simulink model "dog_x_bit_true_2023a1"  (R2023b)
settings: Solver=ode45  StartTime=0.0  StopTime=1.5*lsim*Ts  MaxStep=1/f0/2  RelTol=1e-6
values from neighbouring files (symbols this model uses):
  ft = (bint-1)*fbin    [exe_DOG_X_bit_true_2023a.m]    (also in exe_DOG_X_integer_true_two_paths_5b.m)
  g1 = g1_ideal*1    (= 4)    [exe_DOG_X_bit_true_2023a.m]    (also in exe_DOG_X_integer_true_two_paths_5b.m)
  Kvco = f0    (= 99840000)    [exe_DOG_X_bit_true_2023a.m]    (also in exe_DOG_X_integer_true_two_paths_5b.m)
  lvl = Vfs*10^(Input_signal_dB/20)    (= 0.242661009508)    [exe_DOG_X_bit_true_2023a.m]    (also in exe_DOG_X_integer_true_two_paths_5b.m = 0.125892541179)
  Nbsv1 = Nbvco+4    (= 9)    [exe_DOG_X_bit_true_2023a.m]    (also in exe_DOG_X_integer_true_two_paths_5b.m)
  Nbsv2 = Nbsv1+Nbext    [exe_DOG_X_bit_true_2023a.m]    (also in exe_DOG_X_integer_true_two_paths_5b.m)
  pnoi = 10^(-(60)/10)*(Vfs^2/2)    (= 5e-07)    [exe_DOG_X_bit_true_2023a.m]    (also in exe_DOG_X_integer_true_two_paths_5b.m)
  T2 = 1/f2    (= 4.06901041667e-08)    [exe_DOG_X_bit_true_2023a.m]    (also in exe_DOG_X_integer_true_two_paths_5b.m)
  Ts = 1/fs    (= 3.25520833333e-07)    [exe_DOG_X_bit_true_2023a.m]    (also in exe_DOG_X_integer_true_two_paths_5b.m)
  Vfs = 1    [exe_DOG_X_bit_true_2023a.m]    (also in exe_DOG_X_integer_true_two_paths_5b.m)
undefined symbols (not defined in the file or in its folder): fa, fb
libraries: simulink_extras x86, simulink x8
(part 1 of 4)
settings Model: SimulationMode=accelerator  Creator=lhernandez  LastModifiedBy=Richi
settings DataIOCC: SaveOutput=off  SignalLogging=off  DSMLogging=off  SaveTime=off  ReturnWorkspaceOutputs=off

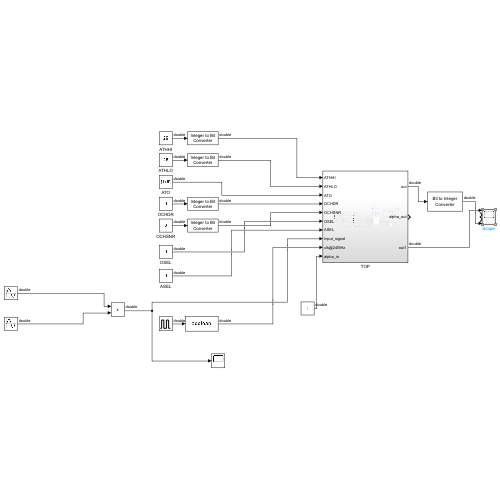
[thumbnail: Simulink's stored preview of the top-level diagram]
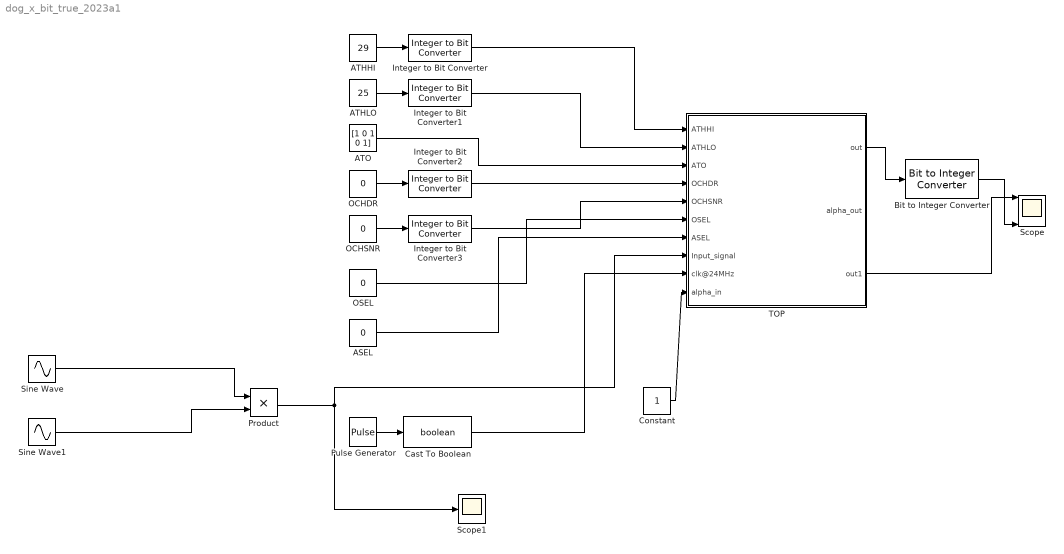
== system dog_x_bit_true_2023a1 ==
  ASEL : Constant  Value=0  OutDataTypeStr=boolean
  ATHHI : Constant  Value=29  OutDataTypeStr=fixdt(0,9,0)
  ATHLO : Constant  Value=25  OutDataTypeStr=fixdt(0,9,0)
  ATO : Constant  Value=[1 0 1 0 1]  OutDataTypeStr=boolean
  Bit to Integer Converter : simulink/Logic and Bit Operations/Bit to Integer Converter  nbits=11  bitOrder=MSB first  signedOutputValues=Signed  outDtype=Inherit via internal rule  outDtypeSigned=double
  Cast To Boolean : DataTypeConversion  OutDataTypeStr=boolean  SaturateOnIntegerOverflow=off  RndMeth=Floor
  Constant : Constant  OutDataTypeStr=boolean
  Integer to Bit Converter : simulink/Logic and Bit Operations/Integer to Bit Converter  nbits=9  signedInputValues=Unsigned  bitOrder=MSB first  outDtype=boolean
  Integer to Bit Converter1 : simulink/Logic and Bit Operations/Integer to Bit Converter  nbits=9  signedInputValues=Unsigned  bitOrder=MSB first  outDtype=boolean
  Integer to Bit Converter2 : simulink/Logic and Bit Operations/Integer to Bit Converter  nbits=4  signedInputValues=Signed  bitOrder=MSB first  outDtype=boolean
  Integer to Bit Converter3 : simulink/Logic and Bit Operations/Integer to Bit Converter  nbits=4  signedInputValues=Signed  bitOrder=MSB first  outDtype=boolean
  OCHDR : Constant  Value=0  OutDataTypeStr=fixdt(1,9,0)
  OCHSNR : Constant  Value=0  OutDataTypeStr=fixdt(1,9,0)
  OSEL : Constant  Value=0  OutDataTypeStr=boolean
  Product : Product
  Pulse Generator : DiscretePulseGenerator  PulseType=Time based  Period=T2  PulseWidth=50
  Scope : Scope  NumInputPorts=4
  Scope1 : Scope
  Sine Wave : Sin  Amplitude=lvl/Vfs  Frequency=2*pi*ft  SampleTime=0
  Sine Wave1 : Sin  Frequency=2*pi*250  SampleTime=0
  TOP : Subsystem
  wires:
  ATHHI/1 -> Integer to Bit Converter/1
  Integer to Bit Converter/1 -> TOP/1(ATHHI)
  ATHLO/1 -> Integer to Bit Converter1/1
  Integer to Bit Converter1/1 -> TOP/2(ATHLO)
  ATO/1 -> TOP/3(ATO)
  OCHDR/1 -> Integer to Bit Converter2/1
  Integer to Bit Converter2/1 -> TOP/4(OCHDR)
  OCHSNR/1 -> Integer to Bit Converter3/1
  Integer to Bit Converter3/1 -> TOP/5(OCHSNR)
  OSEL/1 -> TOP/6(OSEL)
  TOP/1(out) -> Bit to Integer Converter/1
  Pulse Generator/1 -> Cast To Boolean/1
  Cast To Boolean/1 -> TOP/9(clk@24MHz)
  ASEL/1 -> TOP/7(ASEL)
  Sine Wave1/1 -> Product/2
  Sine Wave/1 -> Product/1
  Product/1 -> TOP/8(Input_signal), Scope1/1
  Bit to Integer Converter/1 -> Scope/4
  Constant/1 -> TOP/10(alpha_in)
  TOP/3(out1) -> Scope/1

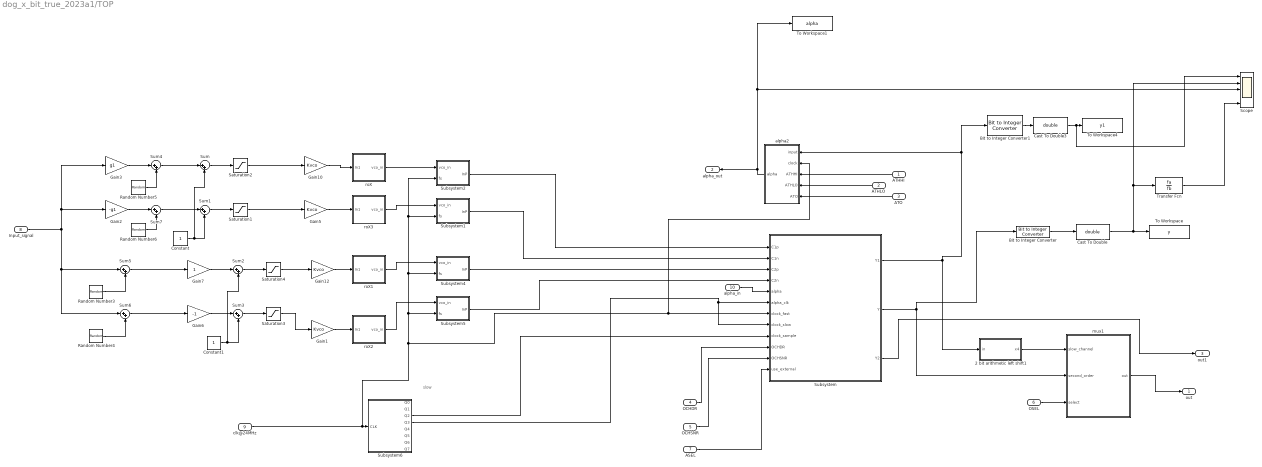
== system dog_x_bit_true_2023a1/TOP ==
  note: slow
  ATHHI : Inport
  ATHLO : Inport  Port=2
  ATO : Inport  Port=3
  OCHDR : Inport  Port=4
  OCHSNR : Inport  Port=5
  OSEL : Inport  Port=6
  ASEL : Inport  Port=7
  Input_signal : Inport  Port=8
  clk@24MHz : Inport  Port=9
  alpha_in : Inport  Port=10
  " 2 bit arithmetic left shift1" : Subsystem
  Bit to Integer Converter : simulink/Logic and Bit Operations/Bit to Integer Converter  nbits=11  bitOrder=MSB first  signedOutputValues=Signed  outDtype=Inherit via internal rule  outDtypeSigned=Inherit via internal rule
  Bit to Integer Converter1 : simulink/Logic and Bit Operations/Bit to Integer Converter  nbits=9  bitOrder=MSB first  signedOutputValues=Signed  outDtype=Inherit via internal rule  outDtypeSigned=Inherit via internal rule
  Cast To Double : DataTypeConversion  OutDataTypeStr=double  SaturateOnIntegerOverflow=off  RndMeth=Floor
  Cast To Double3 : DataTypeConversion  OutDataTypeStr=double  SaturateOnIntegerOverflow=off  RndMeth=Floor
  Constant : Constant
  Constant1 : Constant
  Gain{1,5,10,12} (4 alike) : Gain  Gain=Kvco
  Gain2 : Gain  Gain=-g1
  Gain3 : Gain  Gain=g1
  Gain6 : Gain  Gain=-1
  Gain7 : Gain
  Random Number3 : RandomNumber  Variance=pnoi  Seed=35645  SampleTime=0
  Random Number4 : RandomNumber  Variance=pnoi  Seed=6854  SampleTime=0
  Random Number5 : RandomNumber  Variance=pnoi  Seed=5747  SampleTime=0
  Random Number6 : RandomNumber  Variance=pnoi  Seed=254745  SampleTime=0
  Saturation{1..4} (4 alike) : Saturate  UpperLimit=2  LowerLimit=0
  Scope : Scope  NumInputPorts=5
  Subsystem : Subsystem
  Subsystem1 : Subsystem
  Subsystem2 : Subsystem
  Subsystem4 : Subsystem
  Subsystem5 : Subsystem
  Subsystem6 : Subsystem
  Sum{,1..7} (8 alike) : Sum  Inputs=|++
  To Workspace : ToWorkspace  VariableName=y  SampleTime=Ts
  To Workspace1 : ToWorkspace  VariableName=alpha  SampleTime=Ts
  To Workspace4 : ToWorkspace  VariableName=y1  SampleTime=Ts
  Transfer Fcn : TransferFcn  Numerator=fa  Denominator=fb
  alpha2 : Subsystem
  mux1 : Subsystem
  roX : Subsystem
  roX1 : Subsystem
  roX2 : Subsystem
  roX3 : Subsystem
  out : Outport
  alpha_out : Outport  Port=2
  out1 : Outport  Port=3
  wires:
  roX3/1(vco_in) -> Subsystem1/1(vco_in)
  ? -> Scope/4
  roX/1(vco_in) -> Subsystem2/1(vco_in)
  OSEL/1 -> mux1/3(select)
  ATHLO/1 -> alpha2/4(ATHLO)
  Random Number4/1 -> Sum6/2
  Gain7/1 -> Sum2/1
  Random Number6/1 -> Sum7/2
  Bit to Integer Converter1/1 -> Cast To Double3/1
  Random Number3/1 -> Sum5/2
  Cast To Double/1 -> Transfer Fcn/1, Scope/2, To Workspace/1
  Random Number5/1 -> Sum4/2
  Sum4/1 -> Sum/1
  Saturation4/1 -> Gain12/1
  Gain2/1 -> Sum7/1
  clk@24MHz/1 -> alpha2/2(clock), Subsystem/7(clock_fast), Subsystem5/2(fs), Subsystem4/2(fs), Subsystem2/2(fs), Subsystem1/2(fs), Subsystem6/1(CLK)
  Gain10/1 -> roX/1(In1)
  roX1/1(vco_in) -> Subsystem4/1(vco_in)
  Constant/1 -> Sum/2, Sum1/2
  Bit to Integer Converter/1 -> Cast To Double/1
  Gain3/1 -> Sum4/1
  Sum6/1 -> Gain6/1
  Transfer Fcn/1 -> Scope/5
  Gain5/1 -> roX3/1(In1)
  Sum7/1 -> Sum1/1
  roX2/1(vco_in) -> Subsystem5/1(vco_in)
  Sum/1 -> Saturation2/1
  Gain1/1 -> roX2/1(In1)
  Sum2/1 -> Saturation4/1
  mux1/1(out) -> out/1
  Constant1/1 -> Sum2/2, Sum3/2
  Saturation1/1 -> Gain5/1
  Subsystem/2(Y) -> mux1/2(second_order), Bit to Integer Converter/1
  Saturation3/1 -> Gain1/1
  Saturation2/1 -> Gain10/1
  Gain12/1 -> roX1/1(In1)
  alpha2/1(alpha) -> alpha_out/1, To Workspace1/1, Scope/3
  Cast To Double3/1 -> Scope/1, To Workspace4/1
  Gain6/1 -> Sum3/1
  Sum5/1 -> Gain7/1
  Subsystem/1(Y1) -> " 2 bit arithmetic left shift1"/1(in), Bit to Integer Converter1/1, alpha2/1(input)
  ATHHI/1 -> alpha2/3(ATHHI)
  Input_signal/1 -> Sum6/1, Sum5/1, Gain3/1, Gain2/1
  OCHSNR/1 -> Subsystem/11(OCHSNR)
  Sum3/1 -> Saturation3/1
  Sum1/1 -> Saturation1/1
  ATO/1 -> alpha2/5(ATO)
  OCHDR/1 -> Subsystem/10(OCHDR)
  " 2 bit arithmetic left shift1"/1(x4) -> mux1/1(slow_channel)
  Subsystem2/1(InP) -> Subsystem/1(C1p)
  Subsystem1/1(InP) -> Subsystem/2(C1n)
  Subsystem4/1(InP) -> Subsystem/3(C2p)
  Subsystem5/1(InP) -> Subsystem/4(C2n)
  Subsystem6/4(Q3) -> Subsystem/8(clock_slow), Subsystem/6(alpha_clk)
  Subsystem6/3(Q2) -> Subsystem/9(clock_sample)
  alpha_in/1 -> Subsystem/5(alpha)
  ASEL/1 -> Subsystem/12(use_external)
  Subsystem/3(Y2) -> out1/1

== system dog_x_bit_true_2023a1/TOP/ 2 bit arithmetic left shift1 ==
  in : Inport
  Constant : Constant  Value=0  OutDataTypeStr=boolean
  Demux1 : Demux  Outputs=9
  Mux : Mux  Inputs=11
  x4 : Outport
  wires:
  Mux/1 -> x4/1
  in/1 -> Demux1/1
  Demux1/1 -> Mux/1
  Demux1/2 -> Mux/2
  Demux1/3 -> Mux/3
  Demux1/4 -> Mux/4
  Demux1/5 -> Mux/5
  Demux1/6 -> Mux/6
  Demux1/7 -> Mux/7
  Demux1/8 -> Mux/8
  Demux1/9 -> Mux/9
  Constant/1 -> Mux/11, Mux/10

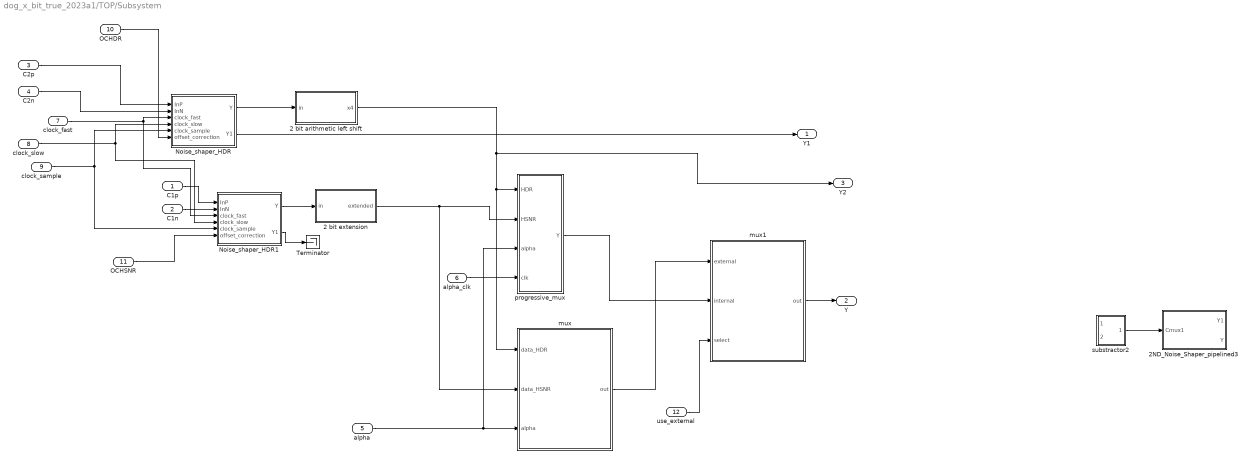
== system dog_x_bit_true_2023a1/TOP/Subsystem ==
  C1p : Inport
  C1n : Inport  Port=2
  C2p : Inport  Port=3
  C2n : Inport  Port=4
  alpha : Inport  Port=5
  alpha_clk : Inport  Port=6
  clock_fast : Inport  Port=7
  clock_slow : Inport  Port=8
  clock_sample : Inport  Port=9
  OCHDR : Inport  Port=10
  OCHSNR : Inport  Port=11
  use_external : Inport  Port=12
  " 2 bit arithmetic left shift" : Subsystem
  " 2 bit extension" : Subsystem
  2ND_Noise_Shaper_pipelined3 : Subsystem
  Noise_shaper_HDR : Subsystem
  Noise_shaper_HDR1 : Subsystem
  Terminator : Terminator
  mux : Subsystem
  mux1 : Subsystem
  progressive_mux : Subsystem
  substractor2 : Subsystem
  Y1 : Outport
  Y : Outport  Port=2
  Y2 : Outport  Port=3
  wires:
  substractor2/1(Cmux1) -> 2ND_Noise_Shaper_pipelined3/1(Cmux1)
  C2p/1 -> Noise_shaper_HDR/1(InP)
  C2n/1 -> Noise_shaper_HDR/2(InN)
  alpha_clk/1 -> progressive_mux/4(clk)
  clock_fast/1 -> Noise_shaper_HDR1/3(clock_fast), Noise_shaper_HDR/3(clock_fast)
  clock_slow/1 -> Noise_shaper_HDR1/4(clock_slow), Noise_shaper_HDR/4(clock_slow)
  Noise_shaper_HDR/1(Y) -> " 2 bit arithmetic left shift"/1(in)
  " 2 bit arithmetic left shift"/1(x4) -> Y2/1, progressive_mux/1(HDR), mux/1(data_HDR)
  clock_sample/1 -> Noise_shaper_HDR1/5(clock_sample), Noise_shaper_HDR/5(clock_sample)
  " 2 bit extension"/1(extended) -> progressive_mux/2(HSNR), mux/2(data_HSNR)
  C1n/1 -> Noise_shaper_HDR1/2(InN)
  C1p/1 -> Noise_shaper_HDR1/1(InP)
  Noise_shaper_HDR1/1(Y) -> " 2 bit extension"/1(in)
  Noise_shaper_HDR1/2(Y1) -> Terminator/1
  mux1/1(out) -> Y/1
  Noise_shaper_HDR/2(Y1) -> Y1/1
  use_external/1 -> mux1/3(select)
  mux/1(out) -> mux1/1(external)
  progressive_mux/1(Y) -> mux1/2(internal)
  alpha/1 -> progressive_mux/3(alpha), mux/3(alpha)
  OCHSNR/1 -> Noise_shaper_HDR1/6(offset_correction)
  OCHDR/1 -> Noise_shaper_HDR/6(offset_correction)

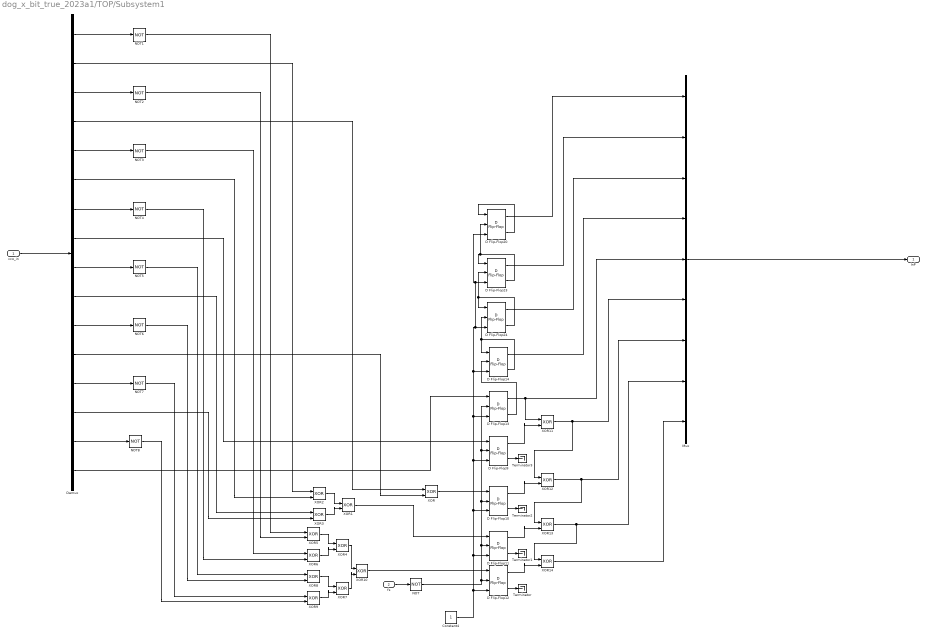
== system dog_x_bit_true_2023a1/TOP/Subsystem1 ==
  vco_in : Inport
  fs : Inport  Port=2
  Constant4 : Constant
  D Flip-Flop{9..14,20,23..24} (9 alike) : simulink_extras/Flip Flops/D Flip-Flop
  Demux : Demux  Outputs=16
  Mux : Mux  Inputs=9
  NOT{,1..8} (9 alike) : Logic  Operator=NOT  IconShape=distinctive  AllPortsSameDT=off  OutDataTypeStr=boolean
  Terminator{,1..3} (4 alike) : Terminator
  XOR{,1..14} (15 alike) : Logic  Operator=XOR  IconShape=distinctive  AllPortsSameDT=off  OutDataTypeStr=boolean
  InP : Outport
  wires:
  D Flip-Flop12/2 -> Terminator/1
  D Flip-Flop10/2 -> Terminator2/1
  D Flip-Flop11/2 -> Terminator1/1
  D Flip-Flop23/2 -> D Flip-Flop20/2, D Flip-Flop23/1
  D Flip-Flop24/2 -> D Flip-Flop24/1, D Flip-Flop23/2
  D Flip-Flop20/2 -> D Flip-Flop20/1
  fs/1 -> NOT/1
  D Flip-Flop14/2 -> D Flip-Flop14/1, D Flip-Flop24/2
  Mux/1 -> InP/1
  Constant4/1 -> D Flip-Flop12/3, D Flip-Flop11/3, D Flip-Flop10/3, D Flip-Flop20/3, D Flip-Flop23/3, D Flip-Flop24/3, D Flip-Flop14/3, D Flip-Flop13/3, D Flip-Flop9/3
  D Flip-Flop13/2 -> D Flip-Flop14/2
  NOT/1 -> D Flip-Flop12/2, D Flip-Flop13/2, D Flip-Flop9/2, D Flip-Flop10/2, D Flip-Flop11/2
  D Flip-Flop9/2 -> Terminator3/1
  vco_in/1 -> Demux/1
  Demux/1 -> NOT1/1
  Demux/5 -> NOT3/1
  Demux/7 -> NOT4/1
  Demux/9 -> NOT5/1
  Demux/13 -> NOT7/1
  Demux/15 -> NOT8/1
  Demux/11 -> NOT6/1
  Demux/4 -> XOR/1
  Demux/12 -> XOR/2
  XOR2/1 -> XOR1/1
  XOR3/1 -> XOR1/2
  Demux/2 -> XOR2/1
  Demux/6 -> XOR2/2
  Demux/10 -> XOR3/1
  Demux/14 -> XOR3/2
  XOR5/1 -> XOR4/1
  XOR6/1 -> XOR4/2
  XOR8/1 -> XOR7/1
  XOR9/1 -> XOR7/2
  XOR4/1 -> XOR10/1
  XOR7/1 -> XOR10/2
  Demux/3 -> NOT2/1
  D Flip-Flop13/1 -> Mux/5, XOR11/1
  D Flip-Flop9/1 -> XOR11/2
  XOR11/1 -> Mux/6, XOR12/1
  D Flip-Flop10/1 -> XOR12/2
  XOR12/1 -> Mux/7, XOR13/1
  D Flip-Flop11/1 -> XOR13/2
  XOR13/1 -> Mux/8, XOR14/1
  D Flip-Flop12/1 -> XOR14/2
  NOT1/1 -> XOR5/1
  NOT2/1 -> XOR5/2
  NOT3/1 -> XOR6/1
  NOT4/1 -> XOR6/2
  NOT5/1 -> XOR8/1
  NOT6/1 -> XOR8/2
  NOT7/1 -> XOR9/1
  NOT8/1 -> XOR9/2
  Demux/16 -> D Flip-Flop13/1
  Demux/8 -> D Flip-Flop9/1
  XOR/1 -> D Flip-Flop10/1
  XOR1/1 -> D Flip-Flop11/1
  XOR10/1 -> D Flip-Flop12/1
  XOR14/1 -> Mux/9
  D Flip-Flop14/1 -> Mux/4
  D Flip-Flop24/1 -> Mux/3
  D Flip-Flop23/1 -> Mux/2
  D Flip-Flop20/1 -> Mux/1

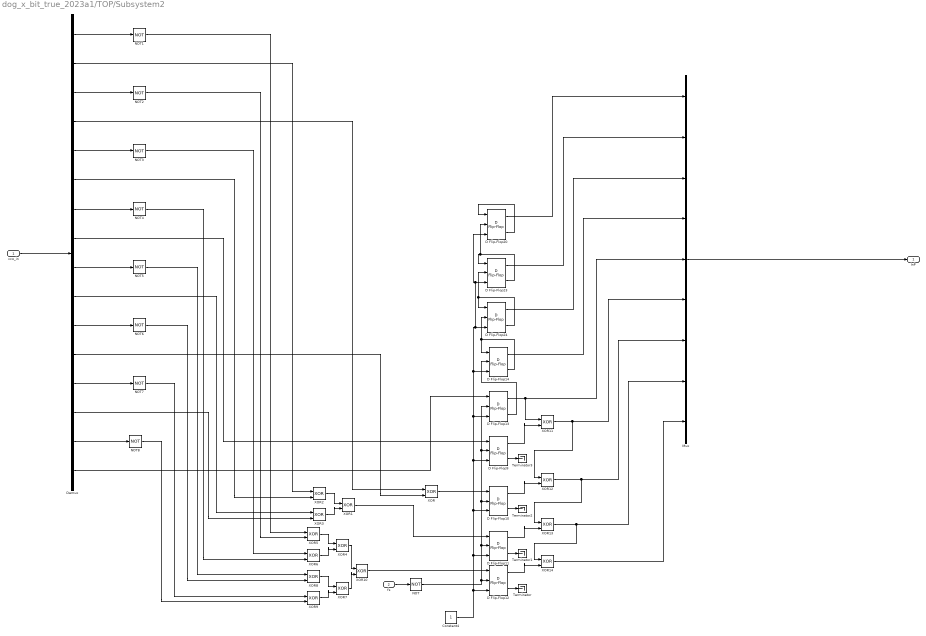
== system dog_x_bit_true_2023a1/TOP/Subsystem2 ==
  vco_in : Inport
  fs : Inport  Port=2
  Constant4 : Constant
  D Flip-Flop{9..14,20,23..24} (9 alike) : simulink_extras/Flip Flops/D Flip-Flop
  Demux : Demux  Outputs=16
  Mux : Mux  Inputs=9
  NOT{,1..8} (9 alike) : Logic  Operator=NOT  IconShape=distinctive  AllPortsSameDT=off  OutDataTypeStr=boolean
  Terminator{,1..3} (4 alike) : Terminator
  XOR{,1..14} (15 alike) : Logic  Operator=XOR  IconShape=distinctive  AllPortsSameDT=off  OutDataTypeStr=boolean
  InP : Outport
  wires:
  D Flip-Flop12/2 -> Terminator/1
  D Flip-Flop10/2 -> Terminator2/1
  D Flip-Flop11/2 -> Terminator1/1
  D Flip-Flop23/2 -> D Flip-Flop20/2, D Flip-Flop23/1
  D Flip-Flop24/2 -> D Flip-Flop24/1, D Flip-Flop23/2
  D Flip-Flop20/2 -> D Flip-Flop20/1
  fs/1 -> NOT/1
  D Flip-Flop14/2 -> D Flip-Flop14/1, D Flip-Flop24/2
  Mux/1 -> InP/1
  Constant4/1 -> D Flip-Flop12/3, D Flip-Flop11/3, D Flip-Flop10/3, D Flip-Flop20/3, D Flip-Flop23/3, D Flip-Flop24/3, D Flip-Flop14/3, D Flip-Flop13/3, D Flip-Flop9/3
  D Flip-Flop13/2 -> D Flip-Flop14/2
  NOT/1 -> D Flip-Flop12/2, D Flip-Flop13/2, D Flip-Flop9/2, D Flip-Flop10/2, D Flip-Flop11/2
  D Flip-Flop9/2 -> Terminator3/1
  vco_in/1 -> Demux/1
  Demux/1 -> NOT1/1
  Demux/5 -> NOT3/1
  Demux/7 -> NOT4/1
  Demux/9 -> NOT5/1
  Demux/13 -> NOT7/1
  Demux/15 -> NOT8/1
  Demux/11 -> NOT6/1
  Demux/4 -> XOR/1
  Demux/12 -> XOR/2
  XOR2/1 -> XOR1/1
  XOR3/1 -> XOR1/2
  Demux/2 -> XOR2/1
  Demux/6 -> XOR2/2
  Demux/10 -> XOR3/1
  Demux/14 -> XOR3/2
  XOR5/1 -> XOR4/1
  XOR6/1 -> XOR4/2
  XOR8/1 -> XOR7/1
  XOR9/1 -> XOR7/2
  XOR4/1 -> XOR10/1
  XOR7/1 -> XOR10/2
  Demux/3 -> NOT2/1
  D Flip-Flop13/1 -> Mux/5, XOR11/1
  D Flip-Flop9/1 -> XOR11/2
  XOR11/1 -> Mux/6, XOR12/1
  D Flip-Flop10/1 -> XOR12/2
  XOR12/1 -> Mux/7, XOR13/1
  D Flip-Flop11/1 -> XOR13/2
  XOR13/1 -> Mux/8, XOR14/1
  D Flip-Flop12/1 -> XOR14/2
  NOT1/1 -> XOR5/1
  NOT2/1 -> XOR5/2
  NOT3/1 -> XOR6/1
  NOT4/1 -> XOR6/2
  NOT5/1 -> XOR8/1
  NOT6/1 -> XOR8/2
  NOT7/1 -> XOR9/1
  NOT8/1 -> XOR9/2
  Demux/16 -> D Flip-Flop13/1
  Demux/8 -> D Flip-Flop9/1
  XOR/1 -> D Flip-Flop10/1
  XOR1/1 -> D Flip-Flop11/1
  XOR10/1 -> D Flip-Flop12/1
  XOR14/1 -> Mux/9
  D Flip-Flop14/1 -> Mux/4
  D Flip-Flop24/1 -> Mux/3
  D Flip-Flop23/1 -> Mux/2
  D Flip-Flop20/1 -> Mux/1

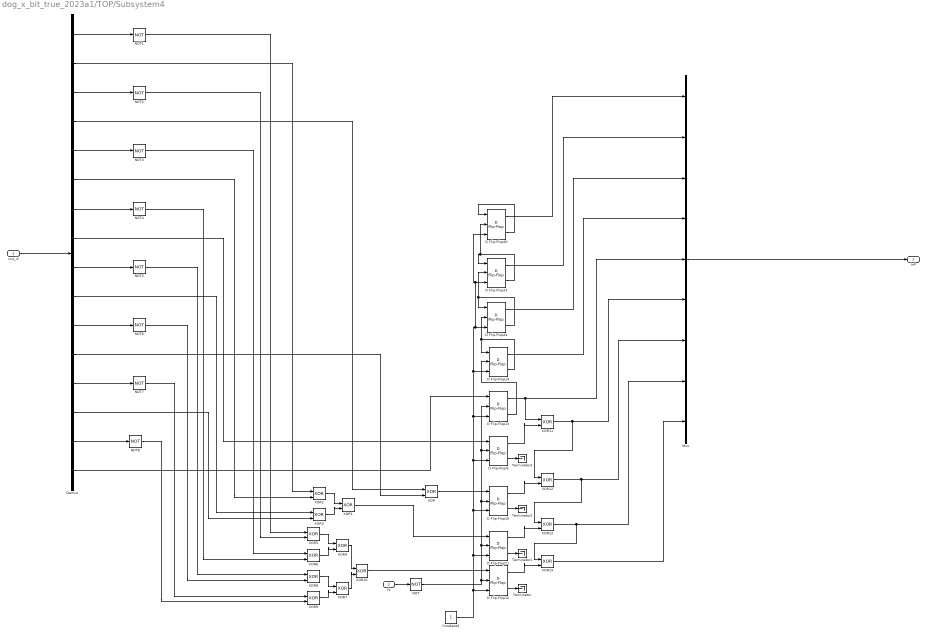
== system dog_x_bit_true_2023a1/TOP/Subsystem4 ==
  vco_in : Inport
  fs : Inport  Port=2
  Constant4 : Constant
  D Flip-Flop{9..14,20,23..24} (9 alike) : simulink_extras/Flip Flops/D Flip-Flop
  Demux : Demux  Outputs=16
  Mux : Mux  Inputs=9
  NOT{,1..8} (9 alike) : Logic  Operator=NOT  IconShape=distinctive  AllPortsSameDT=off  OutDataTypeStr=boolean
  Terminator{,1..3} (4 alike) : Terminator
  XOR{,1..14} (15 alike) : Logic  Operator=XOR  IconShape=distinctive  AllPortsSameDT=off  OutDataTypeStr=boolean
  InP : Outport
  wires:
  D Flip-Flop12/2 -> Terminator/1
  D Flip-Flop10/2 -> Terminator2/1
  D Flip-Flop11/2 -> Terminator1/1
  D Flip-Flop23/2 -> D Flip-Flop20/2, D Flip-Flop23/1
  D Flip-Flop24/2 -> D Flip-Flop24/1, D Flip-Flop23/2
  D Flip-Flop20/2 -> D Flip-Flop20/1
  fs/1 -> NOT/1
  D Flip-Flop14/2 -> D Flip-Flop14/1, D Flip-Flop24/2
  Mux/1 -> InP/1
  Constant4/1 -> D Flip-Flop12/3, D Flip-Flop11/3, D Flip-Flop10/3, D Flip-Flop20/3, D Flip-Flop23/3, D Flip-Flop24/3, D Flip-Flop14/3, D Flip-Flop13/3, D Flip-Flop9/3
  D Flip-Flop13/2 -> D Flip-Flop14/2
  NOT/1 -> D Flip-Flop12/2, D Flip-Flop13/2, D Flip-Flop9/2, D Flip-Flop10/2, D Flip-Flop11/2
  D Flip-Flop9/2 -> Terminator3/1
  vco_in/1 -> Demux/1
  Demux/1 -> NOT1/1
  Demux/5 -> NOT3/1
  Demux/7 -> NOT4/1
  Demux/9 -> NOT5/1
  Demux/13 -> NOT7/1
  Demux/15 -> NOT8/1
  Demux/11 -> NOT6/1
  Demux/4 -> XOR/1
  Demux/12 -> XOR/2
  XOR2/1 -> XOR1/1
  XOR3/1 -> XOR1/2
  Demux/2 -> XOR2/1
  Demux/6 -> XOR2/2
  Demux/10 -> XOR3/1
  Demux/14 -> XOR3/2
  XOR5/1 -> XOR4/1
  XOR6/1 -> XOR4/2
  XOR8/1 -> XOR7/1
  XOR9/1 -> XOR7/2
  XOR4/1 -> XOR10/1
  XOR7/1 -> XOR10/2
  Demux/3 -> NOT2/1
  D Flip-Flop13/1 -> Mux/5, XOR11/1
  D Flip-Flop9/1 -> XOR11/2
  XOR11/1 -> Mux/6, XOR12/1
  D Flip-Flop10/1 -> XOR12/2
  XOR12/1 -> Mux/7, XOR13/1
  D Flip-Flop11/1 -> XOR13/2
  XOR13/1 -> Mux/8, XOR14/1
  D Flip-Flop12/1 -> XOR14/2
  NOT1/1 -> XOR5/1
  NOT2/1 -> XOR5/2
  NOT3/1 -> XOR6/1
  NOT4/1 -> XOR6/2
  NOT5/1 -> XOR8/1
  NOT6/1 -> XOR8/2
  NOT7/1 -> XOR9/1
  NOT8/1 -> XOR9/2
  Demux/16 -> D Flip-Flop13/1
  Demux/8 -> D Flip-Flop9/1
  XOR/1 -> D Flip-Flop10/1
  XOR1/1 -> D Flip-Flop11/1
  XOR10/1 -> D Flip-Flop12/1
  XOR14/1 -> Mux/9
  D Flip-Flop14/1 -> Mux/4
  D Flip-Flop24/1 -> Mux/3
  D Flip-Flop23/1 -> Mux/2
  D Flip-Flop20/1 -> Mux/1

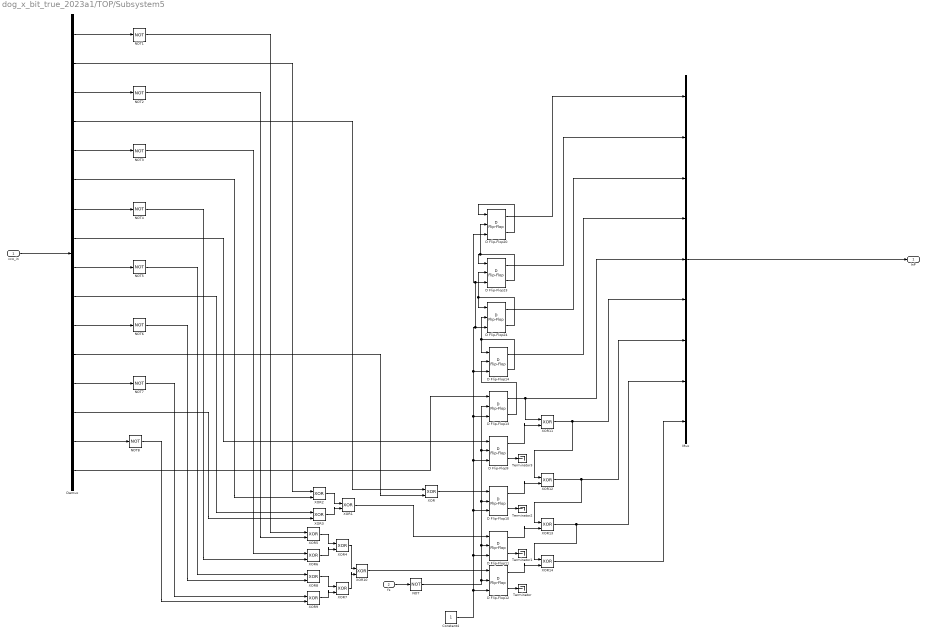
== system dog_x_bit_true_2023a1/TOP/Subsystem5 ==
  vco_in : Inport
  fs : Inport  Port=2
  Constant4 : Constant
  D Flip-Flop{9..14,20,23..24} (9 alike) : simulink_extras/Flip Flops/D Flip-Flop
  Demux : Demux  Outputs=16
  Mux : Mux  Inputs=9
  NOT{,1..8} (9 alike) : Logic  Operator=NOT  IconShape=distinctive  AllPortsSameDT=off  OutDataTypeStr=boolean
  Terminator{,1..3} (4 alike) : Terminator
  XOR{,1..14} (15 alike) : Logic  Operator=XOR  IconShape=distinctive  AllPortsSameDT=off  OutDataTypeStr=boolean
  InP : Outport
  wires:
  D Flip-Flop12/2 -> Terminator/1
  D Flip-Flop10/2 -> Terminator2/1
  D Flip-Flop11/2 -> Terminator1/1
  D Flip-Flop23/2 -> D Flip-Flop20/2, D Flip-Flop23/1
  D Flip-Flop24/2 -> D Flip-Flop24/1, D Flip-Flop23/2
  D Flip-Flop20/2 -> D Flip-Flop20/1
  fs/1 -> NOT/1
  D Flip-Flop14/2 -> D Flip-Flop14/1, D Flip-Flop24/2
  Mux/1 -> InP/1
  Constant4/1 -> D Flip-Flop12/3, D Flip-Flop11/3, D Flip-Flop10/3, D Flip-Flop20/3, D Flip-Flop23/3, D Flip-Flop24/3, D Flip-Flop14/3, D Flip-Flop13/3, D Flip-Flop9/3
  D Flip-Flop13/2 -> D Flip-Flop14/2
  NOT/1 -> D Flip-Flop12/2, D Flip-Flop13/2, D Flip-Flop9/2, D Flip-Flop10/2, D Flip-Flop11/2
  D Flip-Flop9/2 -> Terminator3/1
  vco_in/1 -> Demux/1
  Demux/1 -> NOT1/1
  Demux/5 -> NOT3/1
  Demux/7 -> NOT4/1
  Demux/9 -> NOT5/1
  Demux/13 -> NOT7/1
  Demux/15 -> NOT8/1
  Demux/11 -> NOT6/1
  Demux/4 -> XOR/1
  Demux/12 -> XOR/2
  XOR2/1 -> XOR1/1
  XOR3/1 -> XOR1/2
  Demux/2 -> XOR2/1
  Demux/6 -> XOR2/2
  Demux/10 -> XOR3/1
  Demux/14 -> XOR3/2
  XOR5/1 -> XOR4/1
  XOR6/1 -> XOR4/2
  XOR8/1 -> XOR7/1
  XOR9/1 -> XOR7/2
  XOR4/1 -> XOR10/1
  XOR7/1 -> XOR10/2
  Demux/3 -> NOT2/1
  D Flip-Flop13/1 -> Mux/5, XOR11/1
  D Flip-Flop9/1 -> XOR11/2
  XOR11/1 -> Mux/6, XOR12/1
  D Flip-Flop10/1 -> XOR12/2
  XOR12/1 -> Mux/7, XOR13/1
  D Flip-Flop11/1 -> XOR13/2
  XOR13/1 -> Mux/8, XOR14/1
  D Flip-Flop12/1 -> XOR14/2
  NOT1/1 -> XOR5/1
  NOT2/1 -> XOR5/2
  NOT3/1 -> XOR6/1
  NOT4/1 -> XOR6/2
  NOT5/1 -> XOR8/1
  NOT6/1 -> XOR8/2
  NOT7/1 -> XOR9/1
  NOT8/1 -> XOR9/2
  Demux/16 -> D Flip-Flop13/1
  Demux/8 -> D Flip-Flop9/1
  XOR/1 -> D Flip-Flop10/1
  XOR1/1 -> D Flip-Flop11/1
  XOR10/1 -> D Flip-Flop12/1
  XOR14/1 -> Mux/9
  D Flip-Flop14/1 -> Mux/4
  D Flip-Flop24/1 -> Mux/3
  D Flip-Flop23/1 -> Mux/2
  D Flip-Flop20/1 -> Mux/1

== system dog_x_bit_true_2023a1/TOP/Subsystem6 ==
  CLK : Inport
  Constant2 : Constant
  D Flip-Flop{,1..7} (8 alike) : simulink_extras/Flip Flops/D Flip-Flop
  Q0 : Outport
  Q1 : Outport  Port=2
  Q2 : Outport  Port=3
  Q3 : Outport  Port=4
  Q4 : Outport  Port=5
  Q5 : Outport  Port=6
  Q6 : Outport  Port=7
  Q7 : Outport  Port=8
  wires:
  D Flip-Flop2/2 -> D Flip-Flop3/2, D Flip-Flop2/1
  D Flip-Flop/2 -> D Flip-Flop1/2, D Flip-Flop/1
  D Flip-Flop2/1 -> Q2/1
  D Flip-Flop3/1 -> Q3/1
  D Flip-Flop/1 -> Q0/1
  D Flip-Flop1/1 -> Q1/1
  D Flip-Flop3/2 -> D Flip-Flop3/1, D Flip-Flop4/2
  D Flip-Flop1/2 -> D Flip-Flop2/2, D Flip-Flop1/1
  CLK/1 -> D Flip-Flop/2
  D Flip-Flop5/2 -> D Flip-Flop6/2, D Flip-Flop5/1
  D Flip-Flop4/1 -> Q4/1
  D Flip-Flop5/1 -> Q5/1
  Constant2/1 -> D Flip-Flop1/3, D Flip-Flop2/3, D Flip-Flop3/3, D Flip-Flop4/3, D Flip-Flop5/3, D Flip-Flop6/3, D Flip-Flop7/3, D Flip-Flop/3
  D Flip-Flop6/1 -> Q6/1
  D Flip-Flop7/2 -> D Flip-Flop7/1
  D Flip-Flop6/2 -> D Flip-Flop7/2, D Flip-Flop6/1
  D Flip-Flop7/1 -> Q7/1
  D Flip-Flop4/2 -> D Flip-Flop5/2, D Flip-Flop4/1

== system dog_x_bit_true_2023a1/TOP/alpha2 ==
  note: si a > b, reset
  note: si a > b, HDR
  input : Inport
  clock : Inport  Port=2
  ATHHI : Inport  Port=3
  ATHLO : Inport  Port=4
  ATO : Inport  Port=5
  10 bit  counter (pos) : Subsystem
  AND : Logic  IconShape=distinctive  AllPortsSameDT=off  OutDataTypeStr=boolean
  AND1 : Logic  IconShape=distinctive  AllPortsSameDT=off  OutDataTypeStr=boolean
  NOT : Logic  Operator=NOT  IconShape=distinctive  AllPortsSameDT=off  OutDataTypeStr=boolean
  NOT1 : Logic  Operator=NOT  IconShape=distinctive  AllPortsSameDT=off  OutDataTypeStr=boolean
  NOT2 : Logic  Operator=NOT  IconShape=distinctive  AllPortsSameDT=off  OutDataTypeStr=boolean
  S-R Flip-Flop : simulink_extras/Flip Flops/S-R Flip-Flop  initial_condition=0
  Terminator : Terminator
  abs : Subsystem
  comp_HI_Threshold : Subsystem
  comp_LOW_Threshold : Subsystem
  alpha : Outport
  wires:
  input/1 -> abs/1(input)
  S-R Flip-Flop/1 -> alpha/1
  clock/1 -> 10 bit  counter (pos)/2(clock)
  ATHLO/1 -> comp_LOW_Threshold/2(b)
  NOT1/1 -> 10 bit  counter (pos)/3(!reset)
  abs/1(abs(input)) -> comp_HI_Threshold/1(a), comp_LOW_Threshold/1(a)
  ATHHI/1 -> comp_HI_Threshold/2(b)
  S-R Flip-Flop/2 -> Terminator/1
  comp_LOW_Threshold/1(a < b) -> AND/2
  AND1/1 -> S-R Flip-Flop/2
  comp_HI_Threshold/1(a > b) -> NOT1/1, NOT2/1, S-R Flip-Flop/1
  NOT/1 -> AND/1
  NOT2/1 -> AND1/1
  10 bit  counter (pos)/1(count_selected_bit) -> AND1/2, NOT/1
  AND/1 -> 10 bit  counter (pos)/1(count_enable)
  ATO/1 -> 10 bit  counter (pos)/4(bit_select_mask)

== system dog_x_bit_true_2023a1/TOP/mux1 ==
  slow_channel : Inport
  second_order : Inport  Port=2
  select : Inport  Port=3
  Demux : Demux  Outputs=11
  Demux1 : Demux  Outputs=11
  Mux : Mux  Inputs=11
  Switch{,1..10} (11 alike) : Switch  Criteria=u2 > Threshold  SaturateOnIntegerOverflow=off  InputSameDT=off
  out : Outport
  wires:
  select/1 -> Switch1/2, Switch2/2, Switch3/2, Switch4/2, Switch6/2, Switch7/2, Switch8/2, Switch9/2, Switch10/2, Switch5/2, Switch/2
  slow_channel/1 -> Demux/1
  second_order/1 -> Demux1/1
  Demux/1 -> Switch/1
  Mux/1 -> out/1
  Demux/2 -> Switch1/1
  Demux/3 -> Switch2/1
  Demux/4 -> Switch3/1
  Demux/5 -> Switch4/1
  Demux/6 -> Switch5/1
  Demux/7 -> Switch6/1
  Demux/8 -> Switch7/1
  Demux/9 -> Switch8/1
  Demux/10 -> Switch9/1
  Demux/11 -> Switch10/1
  Demux1/1 -> Switch/3
  Demux1/2 -> Switch1/3
  Demux1/3 -> Switch2/3
  Demux1/4 -> Switch3/3
  Demux1/5 -> Switch4/3
  Demux1/6 -> Switch5/3
  Demux1/7 -> Switch6/3
  Demux1/8 -> Switch7/3
  Demux1/9 -> Switch8/3
  Demux1/10 -> Switch9/3
  Demux1/11 -> Switch10/3
  Switch/1 -> Mux/1
  Switch1/1 -> Mux/2
  Switch2/1 -> Mux/3
  Switch3/1 -> Mux/4
  Switch4/1 -> Mux/5
  Switch5/1 -> Mux/6
  Switch6/1 -> Mux/7
  Switch7/1 -> Mux/8
  Switch8/1 -> Mux/9
  Switch9/1 -> Mux/10
  Switch10/1 -> Mux/11

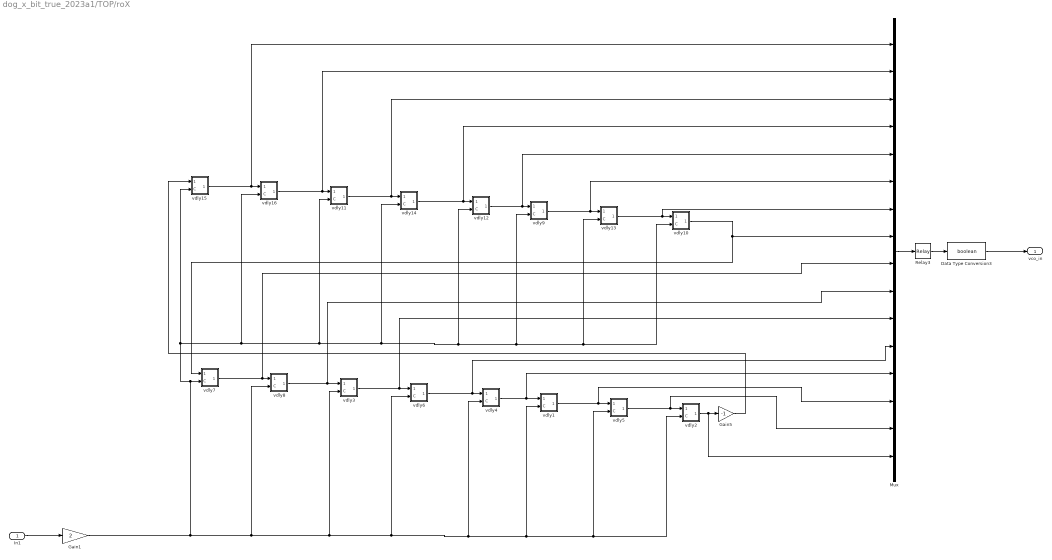
== system dog_x_bit_true_2023a1/TOP/roX ==
  In1 : Inport
  Data Type Conversion3 : DataTypeConversion  OutDataTypeStr=boolean  SaturateOnIntegerOverflow=off  RndMeth=Floor
  Gain1 : Gain  Gain=2
  Gain5 : Gain  Gain=-1
  Mux : Mux  Inputs=16
  Relay3 : Relay
  vdly1 : Subsystem
  vdly10 : Subsystem
  vdly11 : Subsystem
  vdly12 : Subsystem
  vdly13 : Subsystem
  vdly14 : Subsystem
  vdly15 : Subsystem
  vdly16 : Subsystem
  vdly2 : Subsystem
  vdly3 : Subsystem
  vdly4 : Subsystem
  vdly5 : Subsystem
  vdly6 : Subsystem
  vdly7 : Subsystem
  vdly8 : Subsystem
  vdly9 : Subsystem
  vco_in : Outport
  wires:
  vdly2/1(Out) -> Mux/16, Gain5/1
  In1/1 -> Gain1/1
  Gain1/1 -> vdly15/2(C), vdly16/2(C), vdly11/2(C), vdly14/2(C), vdly12/2(C), vdly9/2(C), vdly10/2(C), vdly13/2(C), vdly7/2(C), vdly8/2(C), vdly3/2(C), vdly6/2(C), vdly4/2(C), vdly1/2(C), vdly2/2(C), vdly5/2(C)
  Gain5/1 -> vdly15/1(In)
  Mux/1 -> Relay3/1
  Relay3/1 -> Data Type Conversion3/1
  Data Type Conversion3/1 -> vco_in/1
  vdly5/1(Out) -> Mux/15, vdly2/1(In)
  vdly1/1(Out) -> Mux/14, vdly5/1(In)
  vdly4/1(Out) -> Mux/13, vdly1/1(In)
  vdly6/1(Out) -> Mux/12, vdly4/1(In)
  vdly3/1(Out) -> Mux/11, vdly6/1(In)
  vdly8/1(Out) -> Mux/10, vdly3/1(In)
  vdly7/1(Out) -> vdly8/1(In), Mux/9
  vdly15/1(Out) -> Mux/1, vdly16/1(In)
  vdly16/1(Out) -> Mux/2, vdly11/1(In)
  vdly11/1(Out) -> Mux/3, vdly14/1(In)
  vdly14/1(Out) -> Mux/4, vdly12/1(In)
  vdly12/1(Out) -> Mux/5, vdly9/1(In)
  vdly9/1(Out) -> Mux/6, vdly13/1(In)
  vdly13/1(Out) -> Mux/7, vdly10/1(In)
  vdly10/1(Out) -> vdly7/1(In), Mux/8

== system dog_x_bit_true_2023a1/TOP/roX1 ==
  In1 : Inport
  Data Type Conversion3 : DataTypeConversion  OutDataTypeStr=boolean  SaturateOnIntegerOverflow=off  RndMeth=Floor
  Gain1 : Gain  Gain=2
  Gain5 : Gain  Gain=-1
  Mux : Mux  Inputs=16
  Relay3 : Relay
  vdly1 : Subsystem
  vdly10 : Subsystem
  vdly11 : Subsystem
  vdly12 : Subsystem
  vdly13 : Subsystem
  vdly14 : Subsystem
  vdly15 : Subsystem
  vdly16 : Subsystem
  vdly2 : Subsystem
  vdly3 : Subsystem
  vdly4 : Subsystem
  vdly5 : Subsystem
  vdly6 : Subsystem
  vdly7 : Subsystem
  vdly8 : Subsystem
  vdly9 : Subsystem
  vco_in : Outport
  wires:
  vdly2/1(Out) -> Mux/16, Gain5/1
  In1/1 -> Gain1/1
  Gain1/1 -> vdly15/2(C), vdly16/2(C), vdly11/2(C), vdly14/2(C), vdly12/2(C), vdly9/2(C), vdly10/2(C), vdly13/2(C), vdly7/2(C), vdly8/2(C), vdly3/2(C), vdly6/2(C), vdly4/2(C), vdly1/2(C), vdly2/2(C), vdly5/2(C)
  Gain5/1 -> vdly15/1(In)
  Mux/1 -> Relay3/1
  Relay3/1 -> Data Type Conversion3/1
  Data Type Conversion3/1 -> vco_in/1
  vdly5/1(Out) -> Mux/15, vdly2/1(In)
  vdly1/1(Out) -> Mux/14, vdly5/1(In)
  vdly4/1(Out) -> Mux/13, vdly1/1(In)
  vdly6/1(Out) -> Mux/12, vdly4/1(In)
  vdly3/1(Out) -> Mux/11, vdly6/1(In)
  vdly8/1(Out) -> Mux/10, vdly3/1(In)
  vdly7/1(Out) -> vdly8/1(In), Mux/9
  vdly15/1(Out) -> Mux/1, vdly16/1(In)
  vdly16/1(Out) -> Mux/2, vdly11/1(In)
  vdly11/1(Out) -> Mux/3, vdly14/1(In)
  vdly14/1(Out) -> Mux/4, vdly12/1(In)
  vdly12/1(Out) -> Mux/5, vdly9/1(In)
  vdly9/1(Out) -> Mux/6, vdly13/1(In)
  vdly13/1(Out) -> Mux/7, vdly10/1(In)
  vdly10/1(Out) -> vdly7/1(In), Mux/8

== system dog_x_bit_true_2023a1/TOP/roX2 ==
  In1 : Inport
  Data Type Conversion3 : DataTypeConversion  OutDataTypeStr=boolean  SaturateOnIntegerOverflow=off  RndMeth=Floor
  Gain1 : Gain  Gain=2
  Gain5 : Gain  Gain=-1
  Mux : Mux  Inputs=16
  Relay3 : Relay
  vdly1 : Subsystem
  vdly10 : Subsystem
  vdly11 : Subsystem
  vdly12 : Subsystem
  vdly13 : Subsystem
  vdly14 : Subsystem
  vdly15 : Subsystem
  vdly16 : Subsystem
  vdly2 : Subsystem
  vdly3 : Subsystem
  vdly4 : Subsystem
  vdly5 : Subsystem
  vdly6 : Subsystem
  vdly7 : Subsystem
  vdly8 : Subsystem
  vdly9 : Subsystem
  vco_in : Outport
  wires:
  vdly2/1(Out) -> Mux/16, Gain5/1
  In1/1 -> Gain1/1
  Gain1/1 -> vdly15/2(C), vdly16/2(C), vdly11/2(C), vdly14/2(C), vdly12/2(C), vdly9/2(C), vdly10/2(C), vdly13/2(C), vdly7/2(C), vdly8/2(C), vdly3/2(C), vdly6/2(C), vdly4/2(C), vdly1/2(C), vdly2/2(C), vdly5/2(C)
  Gain5/1 -> vdly15/1(In)
  Mux/1 -> Relay3/1
  Relay3/1 -> Data Type Conversion3/1
  Data Type Conversion3/1 -> vco_in/1
  vdly5/1(Out) -> Mux/15, vdly2/1(In)
  vdly1/1(Out) -> Mux/14, vdly5/1(In)
  vdly4/1(Out) -> Mux/13, vdly1/1(In)
  vdly6/1(Out) -> Mux/12, vdly4/1(In)
  vdly3/1(Out) -> Mux/11, vdly6/1(In)
  vdly8/1(Out) -> Mux/10, vdly3/1(In)
  vdly7/1(Out) -> vdly8/1(In), Mux/9
  vdly15/1(Out) -> Mux/1, vdly16/1(In)
  vdly16/1(Out) -> Mux/2, vdly11/1(In)
  vdly11/1(Out) -> Mux/3, vdly14/1(In)
  vdly14/1(Out) -> Mux/4, vdly12/1(In)
  vdly12/1(Out) -> Mux/5, vdly9/1(In)
  vdly9/1(Out) -> Mux/6, vdly13/1(In)
  vdly13/1(Out) -> Mux/7, vdly10/1(In)
  vdly10/1(Out) -> vdly7/1(In), Mux/8

== system dog_x_bit_true_2023a1/TOP/roX3 ==
  In1 : Inport
  Data Type Conversion3 : DataTypeConversion  OutDataTypeStr=boolean  SaturateOnIntegerOverflow=off  RndMeth=Floor
  Gain1 : Gain  Gain=2
  Gain5 : Gain  Gain=-1
  Mux : Mux  Inputs=16
  Relay3 : Relay
  vdly1 : Subsystem
  vdly10 : Subsystem
  vdly11 : Subsystem
  vdly12 : Subsystem
  vdly13 : Subsystem
  vdly14 : Subsystem
  vdly15 : Subsystem
  vdly16 : Subsystem
  vdly2 : Subsystem
  vdly3 : Subsystem
  vdly4 : Subsystem
  vdly5 : Subsystem
  vdly6 : Subsystem
  vdly7 : Subsystem
  vdly8 : Subsystem
  vdly9 : Subsystem
  vco_in : Outport
  wires:
  vdly2/1(Out) -> Mux/16, Gain5/1
  In1/1 -> Gain1/1
  Gain1/1 -> vdly15/2(C), vdly16/2(C), vdly11/2(C), vdly14/2(C), vdly12/2(C), vdly9/2(C), vdly10/2(C), vdly13/2(C), vdly7/2(C), vdly8/2(C), vdly3/2(C), vdly6/2(C), vdly4/2(C), vdly1/2(C), vdly2/2(C), vdly5/2(C)
  Gain5/1 -> vdly15/1(In)
  Mux/1 -> Relay3/1
  Relay3/1 -> Data Type Conversion3/1
  Data Type Conversion3/1 -> vco_in/1
  vdly5/1(Out) -> Mux/15, vdly2/1(In)
  vdly1/1(Out) -> Mux/14, vdly5/1(In)
  vdly4/1(Out) -> Mux/13, vdly1/1(In)
  vdly6/1(Out) -> Mux/12, vdly4/1(In)
  vdly3/1(Out) -> Mux/11, vdly6/1(In)
  vdly8/1(Out) -> Mux/10, vdly3/1(In)
  vdly7/1(Out) -> vdly8/1(In), Mux/9
  vdly15/1(Out) -> Mux/1, vdly16/1(In)
  vdly16/1(Out) -> Mux/2, vdly11/1(In)
  vdly11/1(Out) -> Mux/3, vdly14/1(In)
  vdly14/1(Out) -> Mux/4, vdly12/1(In)
  vdly12/1(Out) -> Mux/5, vdly9/1(In)
  vdly9/1(Out) -> Mux/6, vdly13/1(In)
  vdly13/1(Out) -> Mux/7, vdly10/1(In)
  vdly10/1(Out) -> vdly7/1(In), Mux/8

== system dog_x_bit_true_2023a1/TOP/Subsystem/ 2 bit arithmetic left shift ==
  in : Inport
  Constant : Constant  Value=0  OutDataTypeStr=boolean
  Demux1 : Demux  Outputs=9
  Mux : Mux  Inputs=11
  x4 : Outport
  wires:
  Mux/1 -> x4/1
  in/1 -> Demux1/1
  Demux1/1 -> Mux/1
  Demux1/2 -> Mux/2
  Demux1/3 -> Mux/3
  Demux1/4 -> Mux/4
  Demux1/5 -> Mux/5
  Demux1/6 -> Mux/6
  Demux1/7 -> Mux/7
  Demux1/8 -> Mux/8
  Demux1/9 -> Mux/9
  Constant/1 -> Mux/11, Mux/10

== system dog_x_bit_true_2023a1/TOP/Subsystem/ 2 bit extension ==
  in : Inport
  Demux1 : Demux  Outputs=9
  Mux : Mux  Inputs=11
  extended : Outport
  wires:
  Mux/1 -> extended/1
  in/1 -> Demux1/1
  Demux1/1 -> Mux/3, Mux/2, Mux/1
  Demux1/2 -> Mux/4
  Demux1/3 -> Mux/5
  Demux1/4 -> Mux/6
  Demux1/5 -> Mux/7
  Demux1/6 -> Mux/8
  Demux1/7 -> Mux/9
  Demux1/8 -> Mux/10
  Demux1/9 -> Mux/11

== system dog_x_bit_true_2023a1/TOP/Subsystem/2ND_Noise_Shaper_pipelined3 ==
  note: 1 / (2^n_shift)
  Cmux1 : Inport
  Data Type Conversion1 : DataTypeConversion  OutDataTypeStr=fixdt(1,Nbsv2,0)  SaturateOnIntegerOverflow=off  RndMeth=Floor
  Data Type Conversion2 : DataTypeConversion  OutDataTypeStr=fixdt(1,Nbsv2,0)  SaturateOnIntegerOverflow=off  RndMeth=Floor
  Delay4 : Delay  DelayLength=1  SampleTime=Ts
  Gain11 : Gain  Gain=1/2^(Nbsv2-Nbsv1)  OutDataTypeStr=fixdt(1,Nbsv1,0)
  M3 : Delay  DelayLength=1  SampleTime=T2
  M4 : Delay  DelayLength=1  SampleTime=T2
  M5 : ZeroOrderHold  SampleTime=Ts
  Sum20 : Sum  Inputs=|+-  OutDataTypeStr=fixdt(1,Nbsv1,0)
  Sum22 : Sum  Inputs=|+-  OutDataTypeStr=fixdt(1,Nbsv2,0)
  Sum8 : Sum  Inputs=|++  OutDataTypeStr=fixdt(1,Nbsv2,0)
  Y1 : Outport
  Y : Outport  Port=2
  wires:
  M5/1 -> Gain11/1
  Data Type Conversion2/1 -> M3/1
  M3/1 -> Sum8/1
  Sum20/1 -> Data Type Conversion2/1
  Delay4/1 -> Sum22/2
  Sum8/1 -> M4/1
  M4/1 -> Sum8/2, M5/1
  Cmux1/1 -> Sum20/1
  Gain11/1 -> Data Type Conversion1/1
  Sum22/1 -> Y/1
  Data Type Conversion1/1 -> Sum20/2, Y1/1, Sum22/1, Delay4/1

== system dog_x_bit_true_2023a1/TOP/Subsystem/Noise_shaper_HDR ==
  InP : Inport
  InN : Inport  Port=2
  clock_fast : Inport  Port=3
  clock_slow : Inport  Port=4
  clock_sample : Inport  Port=5
  offset_correction : Inport  Port=6
  " 3 bit arithmetic right shift" : Subsystem
  DCO : Subsystem
  differential substraction (9 bit) : Subsystem
  feedback substraction (9 bit) : Subsystem
  first difference substraction (9 bit) : Subsystem
  first difference substraction (9 bit)2 : Subsystem
  offset correction : Subsystem
  register2 : Subsystem
  register3 : Subsystem
  register4 : Subsystem
  register5 : Subsystem
  Y : Outport
  Y1 : Outport  Port=2
  wires:
  " 3 bit arithmetic right shift"/1(9 MSB) -> register4/2(D)
  register4/1(Q) -> first difference substraction (9 bit)/1(plus), feedback substraction (9 bit)/2(minus), register5/2(D)
  feedback substraction (9 bit)/1(subs) -> DCO/2(control)
  DCO/1(output) -> " 3 bit arithmetic right shift"/1(in)
  clock_fast/1 -> DCO/1(clock)
  clock_slow/1 -> register3/1(CLK), register2/1(CLK)
  register2/1(Q) -> first difference substraction (9 bit)2/1(plus), register3/2(D)
  first difference substraction (9 bit)2/1(subs) -> Y1/1
  InP/1 -> differential substraction (9 bit)/1(counter P)
  InN/1 -> differential substraction (9 bit)/2(conter N)
  clock_sample/1 -> register4/1(CLK), register5/1(CLK)
  register3/1(Q) -> first difference substraction (9 bit)2/2(minus)
  register5/1(Q) -> first difference substraction (9 bit)/2(minus)
  differential substraction (9 bit)/1(subs) -> register2/2(D), feedback substraction (9 bit)/1(plus)
  offset_correction/1 -> offset correction/2(b)
  offset correction/1(sum) -> Y/1
  first difference substraction (9 bit)/1(subs) -> offset correction/1(a)

== system dog_x_bit_true_2023a1/TOP/Subsystem/Noise_shaper_HDR1 ==
  InP : Inport
  InN : Inport  Port=2
  clock_fast : Inport  Port=3
  clock_slow : Inport  Port=4
  clock_sample : Inport  Port=5
  offset_correction : Inport  Port=6
  " 3 bit arithmetic right shift" : Subsystem
  DCO : Subsystem
  differential substraction (9 bit) : Subsystem
  feedback substraction (9 bit) : Subsystem
  first difference substraction (9 bit) : Subsystem
  first difference substraction (9 bit)2 : Subsystem
  offset correction : Subsystem
  register2 : Subsystem
  register3 : Subsystem
  register4 : Subsystem
  register5 : Subsystem
  Y : Outport
  Y1 : Outport  Port=2
  wires:
  " 3 bit arithmetic right shift"/1(9 MSB) -> register4/2(D)
  register4/1(Q) -> first difference substraction (9 bit)/1(plus), feedback substraction (9 bit)/2(minus), register5/2(D)
  feedback substraction (9 bit)/1(subs) -> DCO/2(control)
  DCO/1(output) -> " 3 bit arithmetic right shift"/1(in)
  clock_fast/1 -> DCO/1(clock)
  clock_slow/1 -> register3/1(CLK), register2/1(CLK)
  register2/1(Q) -> first difference substraction (9 bit)2/1(plus), register3/2(D)
  first difference substraction (9 bit)2/1(subs) -> Y1/1
  InP/1 -> differential substraction (9 bit)/1(counter P)
  InN/1 -> differential substraction (9 bit)/2(conter N)
  clock_sample/1 -> register4/1(CLK), register5/1(CLK)
  register3/1(Q) -> first difference substraction (9 bit)2/2(minus)
  register5/1(Q) -> first difference substraction (9 bit)/2(minus)
  differential substraction (9 bit)/1(subs) -> register2/2(D), feedback substraction (9 bit)/1(plus)
  offset_correction/1 -> offset correction/2(b)
  offset correction/1(sum) -> Y/1
  first difference substraction (9 bit)/1(subs) -> offset correction/1(a)

== system dog_x_bit_true_2023a1/TOP/Subsystem/mux ==
  data_HDR : Inport
  data_HSNR : Inport  Port=2
  alpha : Inport  Port=3
  Demux : Demux  Outputs=11
  Demux1 : Demux  Outputs=11
  Mux : Mux  Inputs=11
  Switch{,1..10} (11 alike) : Switch  Criteria=u2 > Threshold  SaturateOnIntegerOverflow=off  InputSameDT=off
  out : Outport
  wires:
  alpha/1 -> Switch1/2, Switch2/2, Switch3/2, Switch4/2, Switch6/2, Switch7/2, Switch8/2, Switch9/2, Switch10/2, Switch5/2, Switch/2
  data_HDR/1 -> Demux/1
  data_HSNR/1 -> Demux1/1
  Demux/1 -> Switch/1
  Mux/1 -> out/1
  Demux/2 -> Switch1/1
  Demux/3 -> Switch2/1
  Demux/4 -> Switch3/1
  Demux/5 -> Switch4/1
  Demux/6 -> Switch5/1
  Demux/7 -> Switch6/1
  Demux/8 -> Switch7/1
  Demux/9 -> Switch8/1
  Demux/10 -> Switch9/1
  Demux/11 -> Switch10/1
  Demux1/1 -> Switch/3
  Demux1/2 -> Switch1/3
  Demux1/3 -> Switch2/3
  Demux1/4 -> Switch3/3
  Demux1/5 -> Switch4/3
  Demux1/6 -> Switch5/3
  Demux1/7 -> Switch6/3
  Demux1/8 -> Switch7/3
  Demux1/9 -> Switch8/3
  Demux1/10 -> Switch9/3
  Demux1/11 -> Switch10/3
  Switch/1 -> Mux/1
  Switch1/1 -> Mux/2
  Switch2/1 -> Mux/3
  Switch3/1 -> Mux/4
  Switch4/1 -> Mux/5
  Switch5/1 -> Mux/6
  Switch6/1 -> Mux/7
  Switch7/1 -> Mux/8
  Switch8/1 -> Mux/9
  Switch9/1 -> Mux/10
  Switch10/1 -> Mux/11

== system dog_x_bit_true_2023a1/TOP/Subsystem/mux1 ==
  external : Inport
  internal : Inport  Port=2
  select : Inport  Port=3
  Demux : Demux  Outputs=11
  Demux1 : Demux  Outputs=11
  Mux : Mux  Inputs=11
  Switch{,1..10} (11 alike) : Switch  Criteria=u2 > Threshold  SaturateOnIntegerOverflow=off  InputSameDT=off
  out : Outport
  wires:
  select/1 -> Switch1/2, Switch2/2, Switch3/2, Switch4/2, Switch6/2, Switch7/2, Switch8/2, Switch9/2, Switch10/2, Switch5/2, Switch/2
  external/1 -> Demux/1
  internal/1 -> Demux1/1
  Demux/1 -> Switch/1
  Mux/1 -> out/1
  Demux/2 -> Switch1/1
  Demux/3 -> Switch2/1
  Demux/4 -> Switch3/1
  Demux/5 -> Switch4/1
  Demux/6 -> Switch5/1
  Demux/7 -> Switch6/1
  Demux/8 -> Switch7/1
  Demux/9 -> Switch8/1
  Demux/10 -> Switch9/1
  Demux/11 -> Switch10/1
  Demux1/1 -> Switch/3
  Demux1/2 -> Switch1/3
  Demux1/3 -> Switch2/3
  Demux1/4 -> Switch3/3
  Demux1/5 -> Switch4/3
  Demux1/6 -> Switch5/3
  Demux1/7 -> Switch6/3
  Demux1/8 -> Switch7/3
  Demux1/9 -> Switch8/3
  Demux1/10 -> Switch9/3
  Demux1/11 -> Switch10/3
  Switch/1 -> Mux/1
  Switch1/1 -> Mux/2
  Switch2/1 -> Mux/3
  Switch3/1 -> Mux/4
  Switch4/1 -> Mux/5
  Switch5/1 -> Mux/6
  Switch6/1 -> Mux/7
  Switch7/1 -> Mux/8
  Switch8/1 -> Mux/9
  Switch9/1 -> Mux/10
  Switch10/1 -> Mux/11

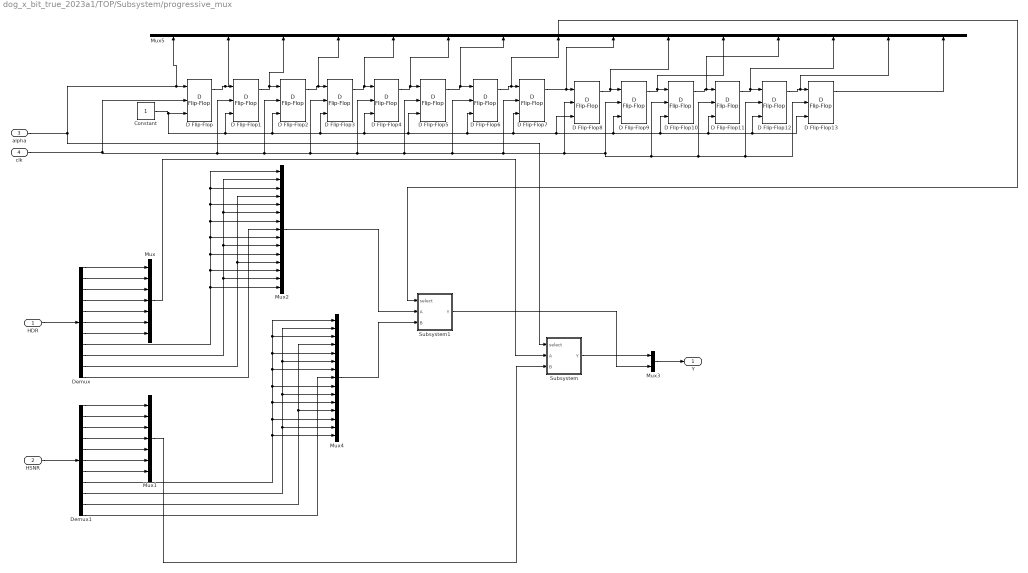
== system dog_x_bit_true_2023a1/TOP/Subsystem/progressive_mux ==
  HDR : Inport
  HSNR : Inport  Port=2
  alpha : Inport  Port=3
  clk : Inport  Port=4
  Constant : Constant  OutDataTypeStr=boolean
  D Flip-Flop{,1..13} (14 alike) : simulink_extras/Flip Flops/D Flip-Flop
  Demux : Demux  Outputs=11
  Demux1 : Demux  Outputs=11
  Mux : Mux  Inputs=7
  Mux1 : Mux  Inputs=7
  Mux2 : Mux  Inputs=15
  Mux3 : Mux  Inputs=2
  Mux4 : Mux  Inputs=15
  Mux5 : Mux  Inputs=15
  Subsystem : Subsystem
  Subsystem1 : Subsystem
  Y : Outport
  wires:
  HSNR/1 -> Demux1/1
  HDR/1 -> Demux/1
  Demux/1 -> Mux/1
  Demux/2 -> Mux/2
  Demux/3 -> Mux/3
  Demux/4 -> Mux/4
  Demux/5 -> Mux/5
  Demux/6 -> Mux/6
  Demux/7 -> Mux/7
  Demux1/5 -> Mux1/5
  Demux1/7 -> Mux1/7
  Demux1/6 -> Mux1/6
  Demux1/4 -> Mux1/4
  Demux1/3 -> Mux1/3
  Demux1/2 -> Mux1/2
  Demux1/1 -> Mux1/1
  D Flip-Flop/1 -> Mux5/2, D Flip-Flop1/1
  D Flip-Flop1/1 -> Mux5/3, D Flip-Flop2/1
  D Flip-Flop4/1 -> Mux5/6, D Flip-Flop5/1
  D Flip-Flop3/1 -> Mux5/5, D Flip-Flop4/1
  D Flip-Flop2/1 -> Mux5/4, D Flip-Flop3/1
  D Flip-Flop7/1 -> Mux5/9, D Flip-Flop8/1
  D Flip-Flop6/1 -> Mux5/8, D Flip-Flop7/1
  D Flip-Flop5/1 -> Mux5/7, D Flip-Flop6/1
  alpha/1 -> Mux5/1, D Flip-Flop/1, Subsystem/1(select)
  Mux3/1 -> Y/1
  Mux/1 -> Subsystem/2(A)
  Mux1/1 -> Subsystem/3(B)
  Subsystem/1(Y) -> Mux3/1
  Mux2/1 -> Subsystem1/2(A)
  Mux4/1 -> Subsystem1/3(B)
  D Flip-Flop9/1 -> Mux5/11, D Flip-Flop10/1
  D Flip-Flop8/1 -> Mux5/10, D Flip-Flop9/1
  Constant/1 -> D Flip-Flop1/3, D Flip-Flop8/3, D Flip-Flop13/3, D Flip-Flop12/3, D Flip-Flop11/3, D Flip-Flop10/3, D Flip-Flop9/3, D Flip-Flop7/3, D Flip-Flop6/3, D Flip-Flop5/3, D Flip-Flop4/3, D Flip-Flop3/3, D Flip-Flop2/3, D Flip-Flop/3
  D Flip-Flop10/1 -> Mux5/12, D Flip-Flop11/1
  D Flip-Flop11/1 -> Mux5/13, D Flip-Flop12/1
  D Flip-Flop12/1 -> Mux5/14, D Flip-Flop13/1
  D Flip-Flop13/1 -> Mux5/15
  clk/1 -> D Flip-Flop6/2, D Flip-Flop7/2, D Flip-Flop8/2, D Flip-Flop9/2, D Flip-Flop10/2, D Flip-Flop13/2, D Flip-Flop12/2, D Flip-Flop11/2, D Flip-Flop5/2, D Flip-Flop4/2, D Flip-Flop3/2, D Flip-Flop2/2, D Flip-Flop1/2, D Flip-Flop/2
  Mux5/1 -> Subsystem1/1(select)
  Subsystem1/1(Y) -> Mux3/2
  Demux/8 -> Mux2/15, Mux2/13, Mux2/11, Mux2/9, Mux2/7, Mux2/5, Mux2/3, Mux2/1
  Demux/9 -> Mux2/14, Mux2/10, Mux2/6, Mux2/2
  Demux/10 -> Mux2/12, Mux2/4
  Demux/11 -> Mux2/8
  Demux1/8 -> Mux4/15, Mux4/13, Mux4/11, Mux4/9, Mux4/7, Mux4/5, Mux4/3, Mux4/1
  Demux1/9 -> Mux4/14, Mux4/10, Mux4/6, Mux4/2
  Demux1/10 -> Mux4/12, Mux4/4
  Demux1/11 -> Mux4/8

== system dog_x_bit_true_2023a1/TOP/Subsystem/substractor2 ==
  note: to 2's comp (NbC1 bits)
  C2p : Inport
  C2n : Inport  Port=2
  Add1 : Sum
  Add2 : Sum
  Constant13 : Constant  Value=-(2^(Nbsv1-1))
  Data Type Conversion : DataTypeConversion  OutDataTypeStr=fixdt(1,Nbsv1,0)  SaturateOnIntegerOverflow=off  RndMeth=Floor
  Data Type Conversion1 : DataTypeConversion  OutDataTypeStr=fixdt(1,Nbsv1,0)  SaturateOnIntegerOverflow=off  RndMeth=Floor
  M2 : Delay  DelayLength=1  SampleTime=T2
  Sum19 : Sum  Inputs=+-  OutDataTypeStr=fixdt(1,Nbsv1,0)
  Cmux1 : Outport
  wires:
  Data Type Conversion1/1 -> Sum19/2
  Add1/1 -> Data Type Conversion/1
  Constant13/1 -> Add2/1, Add1/1
  Data Type Conversion/1 -> Sum19/1
  Sum19/1 -> M2/1
  Add2/1 -> Data Type Conversion1/1
  C2p/1 -> Add1/2
  M2/1 -> Cmux1/1
  C2n/1 -> Add2/2

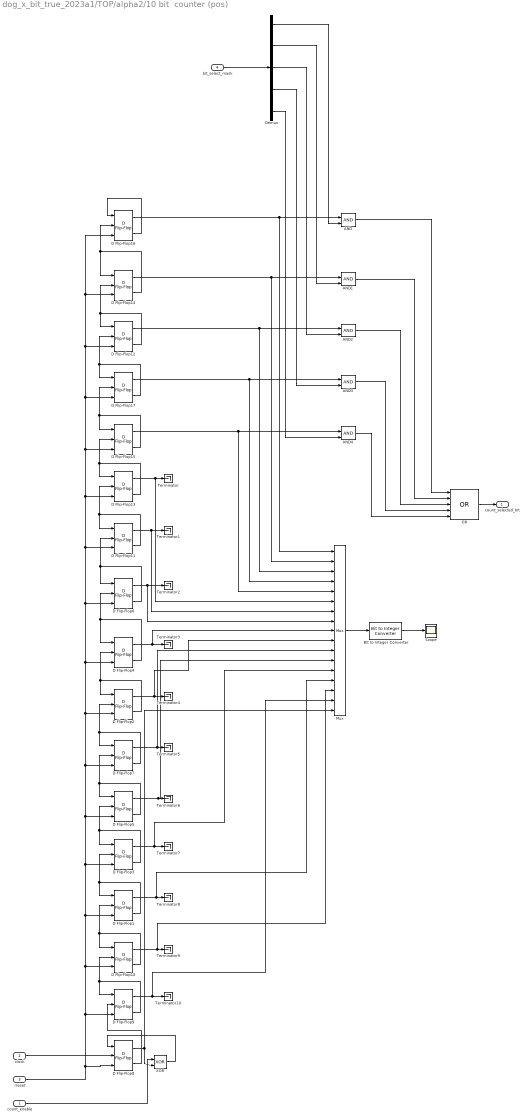
== system dog_x_bit_true_2023a1/TOP/alpha2/10 bit  counter (pos) ==
  count_enable : Inport
  clock : Inport  Port=2
  !reset : Inport  Port=3
  bit_select_mask : Inport  Port=4
  AND{,1..4} (5 alike) : Logic  IconShape=distinctive  AllPortsSameDT=off  OutDataTypeStr=boolean
  Bit to Integer Converter : simulink/Logic and Bit Operations/Bit to Integer Converter  nbits=17  bitOrder=MSB first  signedOutputValues=Unsigned  outDtype=Inherit via internal rule  outDtypeSigned=Inherit via internal rule
  D Flip-Flop{1..17} (17 alike) : simulink_extras/Flip Flops/D Flip-Flop
  Demux : Demux  Outputs=5
  Mux : Mux  Inputs=17
  OR : Logic  Operator=OR  Inputs=5  IconShape=distinctive  AllPortsSameDT=off  OutDataTypeStr=boolean
  Scope : Scope
  Terminator{,1..10} (11 alike) : Terminator
  XOR : Logic  Operator=XOR  IconShape=distinctive  AllPortsSameDT=off  OutDataTypeStr=boolean
  count_selected_bit : Outport
  wires:
  D Flip-Flop1/2 -> D Flip-Flop3/2, D Flip-Flop1/1
  D Flip-Flop3/2 -> D Flip-Flop3/1, D Flip-Flop5/2
  D Flip-Flop5/2 -> D Flip-Flop7/2, D Flip-Flop5/1
  D Flip-Flop7/2 -> D Flip-Flop2/2, D Flip-Flop7/1
  D Flip-Flop2/2 -> D Flip-Flop4/2, D Flip-Flop2/1
  D Flip-Flop6/2 -> D Flip-Flop11/2, D Flip-Flop6/1
  D Flip-Flop9/2 -> D Flip-Flop9/1, D Flip-Flop10/2
  D Flip-Flop10/2 -> D Flip-Flop1/2, D Flip-Flop10/1
  clock/1 -> D Flip-Flop8/2
  D Flip-Flop8/2 -> D Flip-Flop9/2
  count_enable/1 -> XOR/1
  XOR/1 -> D Flip-Flop8/1
  D Flip-Flop8/1 -> Mux/17, XOR/2
  bit_select_mask/1 -> Demux/1
  D Flip-Flop16/1 -> Mux/1, AND/1
  !reset/1 -> D Flip-Flop8/3, D Flip-Flop9/3, D Flip-Flop10/3, D Flip-Flop3/3, D Flip-Flop5/3, D Flip-Flop11/3, D Flip-Flop13/3, D Flip-Flop15/3, D Flip-Flop16/3, D Flip-Flop14/3, D Flip-Flop12/3, D Flip-Flop17/3, D Flip-Flop6/3, D Flip-Flop4/3, D Flip-Flop2/3, D Flip-Flop7/3, D Flip-Flop1/3
  D Flip-Flop11/2 -> D Flip-Flop13/2, D Flip-Flop11/1
  D Flip-Flop4/2 -> D Flip-Flop6/2, D Flip-Flop4/1
  D Flip-Flop15/2 -> D Flip-Flop17/2, D Flip-Flop15/1
  D Flip-Flop15/1 -> Mux/5, AND4/1
  D Flip-Flop12/1 -> Mux/3, AND2/1
  D Flip-Flop16/2 -> D Flip-Flop16/1
  D Flip-Flop17/2 -> D Flip-Flop12/2, D Flip-Flop17/1
  D Flip-Flop12/2 -> D Flip-Flop14/2, D Flip-Flop12/1
  D Flip-Flop14/1 -> Mux/2, AND1/1
  D Flip-Flop14/2 -> D Flip-Flop16/2, D Flip-Flop14/1
  D Flip-Flop17/1 -> Mux/4, AND3/1
  D Flip-Flop13/2 -> D Flip-Flop13/1, D Flip-Flop15/2
  AND/1 -> OR/1
  AND4/1 -> OR/5
  AND1/1 -> OR/2
  AND3/1 -> OR/4
  OR/1 -> count_selected_bit/1
  AND2/1 -> OR/3
  D Flip-Flop13/1 -> Mux/6, Terminator/1
  D Flip-Flop11/1 -> Mux/7, Terminator1/1
  D Flip-Flop4/1 -> Mux/9, Terminator3/1
  D Flip-Flop6/1 -> Mux/8, Terminator2/1
  D Flip-Flop2/1 -> Mux/10, Terminator4/1
  D Flip-Flop7/1 -> Mux/11, Terminator5/1
  D Flip-Flop1/1 -> Mux/14, Terminator8/1
  D Flip-Flop9/1 -> Mux/16, Terminator10/1
  D Flip-Flop3/1 -> Mux/13, Terminator7/1
  D Flip-Flop10/1 -> Mux/15, Terminator9/1
  D Flip-Flop5/1 -> Mux/12, Terminator6/1
  Demux/5 -> AND4/2
  Demux/4 -> AND3/2
  Demux/3 -> AND2/2
  Demux/2 -> AND1/2
  Demux/1 -> AND/2
  Mux/1 -> Bit to Integer Converter/1
  Bit to Integer Converter/1 -> Scope/1

== system dog_x_bit_true_2023a1/TOP/alpha2/abs ==
  input : Inport
  Constant : Constant  OutDataTypeStr=boolean
  Constant2 : Constant  Value=0  OutDataTypeStr=boolean
  Demux1 : Demux  Outputs=9
  FA10 : Subsystem
  FA2 : Subsystem
  FA3 : Subsystem
  FA4 : Subsystem
  FA5 : Subsystem
  FA6 : Subsystem
  FA7 : Subsystem
  FA9 : Subsystem
  Mux : Mux  Inputs=9
  XOR{,1..7} (8 alike) : Logic  Operator=XOR  IconShape=distinctive  AllPortsSameDT=off  OutDataTypeStr=boolean
  abs(input) : Outport
  wires:
  Mux/1 -> abs(input)/1
  input/1 -> Demux1/1
  FA7/2(Co) -> FA6/3(Cin)
  FA6/2(Co) -> FA5/3(Cin)
  FA5/2(Co) -> FA4/3(Cin)
  FA4/2(Co) -> FA3/3(Cin)
  FA3/2(Co) -> FA2/3(Cin)
  FA9/2(Co) -> FA7/3(Cin)
  FA10/2(Co) -> FA9/2(Cin)
  Constant/1 -> FA10/3(Cin)
  FA2/1(S) -> Mux/2
  FA2/2(Co) -> Mux/1
  FA3/1(S) -> Mux/3
  FA4/1(S) -> Mux/4
  FA5/1(S) -> Mux/5
  FA6/1(S) -> Mux/6
  FA7/1(S) -> Mux/7
  FA9/1(S) -> Mux/8
  FA10/1(S) -> Mux/9
  XOR/1 -> FA2/1(B0)
  Constant2/1 -> FA5/2(B1), FA6/2(B1), FA9/3(B1), FA10/2(B1), FA7/2(B1), FA4/2(B1), FA3/2(B1), FA2/2(B1)
  XOR1/1 -> FA3/1(B0)
  XOR2/1 -> FA4/1(B0)
  XOR3/1 -> FA5/1(B0)
  XOR4/1 -> FA6/1(B0)
  XOR5/1 -> FA7/1(B0)
  XOR6/1 -> FA9/1(B0)
  XOR7/1 -> FA10/1(B0)
  Demux1/1 -> XOR1/1, XOR3/1, XOR4/1, XOR5/1, XOR6/1, XOR7/1, XOR2/1, XOR/1
  Demux1/2 -> XOR/2
  Demux1/3 -> XOR1/2
  Demux1/4 -> XOR2/2
  Demux1/5 -> XOR3/2
  Demux1/6 -> XOR4/2
  Demux1/7 -> XOR5/2
  Demux1/8 -> XOR6/2
  Demux1/9 -> XOR7/2

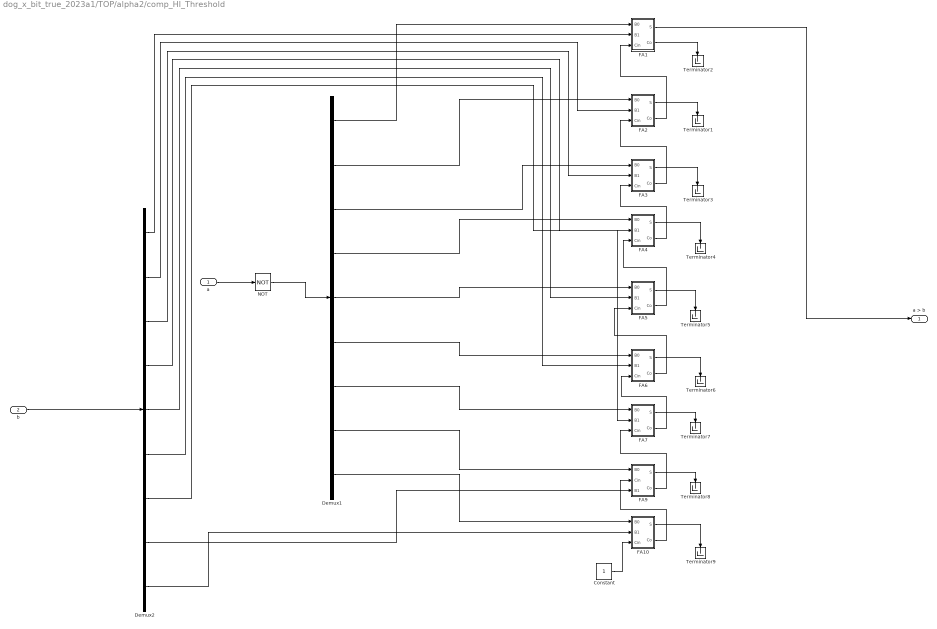
== system dog_x_bit_true_2023a1/TOP/alpha2/comp_HI_Threshold ==
  a : Inport
  b : Inport  Port=2
  Constant : Constant  OutDataTypeStr=boolean
  Demux1 : Demux  Outputs=9
  Demux2 : Demux  Outputs=9
  FA1 : Subsystem
  FA10 : Subsystem
  FA2 : Subsystem
  FA3 : Subsystem
  FA4 : Subsystem
  FA5 : Subsystem
  FA6 : Subsystem
  FA7 : Subsystem
  FA9 : Subsystem
  NOT : Logic  Operator=NOT  IconShape=distinctive  AllPortsSameDT=off  OutDataTypeStr=boolean
  Terminator{1..9} (9 alike) : Terminator
  a > b : Outport
  wires:
  a/1 -> NOT/1
  FA7/2(Co) -> FA6/3(Cin)
  FA6/2(Co) -> FA5/3(Cin)
  FA5/2(Co) -> FA4/3(Cin)
  FA4/2(Co) -> FA3/3(Cin)
  FA3/2(Co) -> FA2/3(Cin)
  FA2/2(Co) -> FA1/3(Cin)
  FA9/2(Co) -> FA7/3(Cin)
  FA10/2(Co) -> FA9/2(Cin)
  Constant/1 -> FA10/3(Cin)
  FA1/2(Co) -> Terminator2/1
  Demux1/9 -> FA10/1(B0)
  Demux1/8 -> FA9/1(B0)
  Demux1/7 -> FA7/1(B0)
  Demux1/6 -> FA6/1(B0)
  Demux1/5 -> FA5/1(B0)
  Demux1/4 -> FA4/1(B0)
  Demux1/2 -> FA2/1(B0)
  Demux1/3 -> FA3/1(B0)
  Demux1/1 -> FA1/1(B0)
  FA1/1(S) -> a > b/1
  Demux2/5 -> FA5/2(B1)
  Demux2/6 -> FA6/2(B1)
  Demux2/1 -> FA1/2(B1)
  Demux2/3 -> FA3/2(B1)
  Demux2/4 -> FA4/2(B1)
  Demux2/2 -> FA2/2(B1)
  Demux2/7 -> FA7/2(B1)
  Demux2/9 -> FA10/2(B1)
  Demux2/8 -> FA9/3(B1)
  FA2/1(S) -> Terminator1/1
  FA3/1(S) -> Terminator3/1
  FA4/1(S) -> Terminator4/1
  FA5/1(S) -> Terminator5/1
  FA6/1(S) -> Terminator6/1
  FA7/1(S) -> Terminator7/1
  FA9/1(S) -> Terminator8/1
  FA10/1(S) -> Terminator9/1
  b/1 -> Demux2/1
  NOT/1 -> Demux1/1

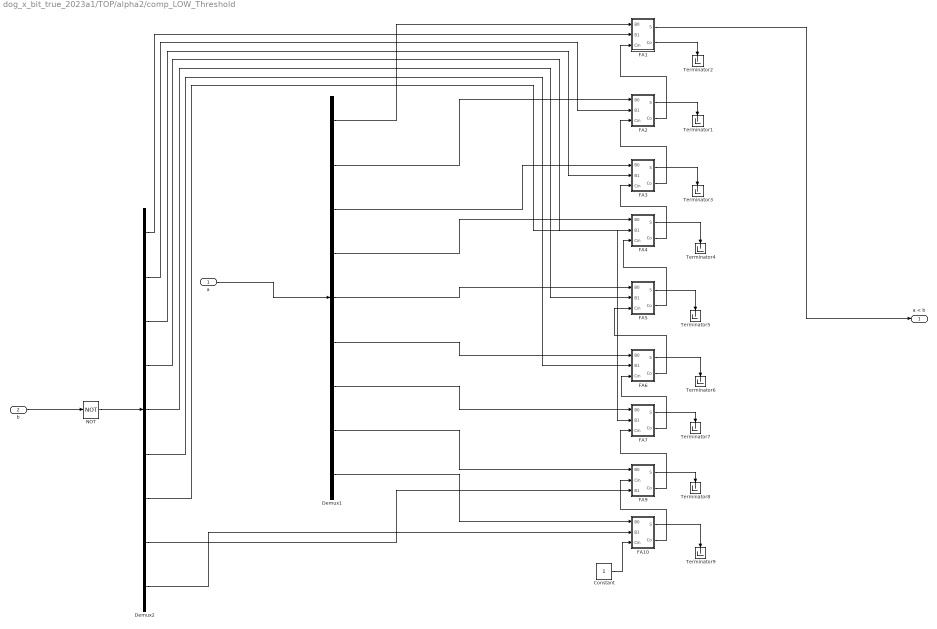
== system dog_x_bit_true_2023a1/TOP/alpha2/comp_LOW_Threshold ==
  a : Inport
  b : Inport  Port=2
  Constant : Constant  OutDataTypeStr=boolean
  Demux1 : Demux  Outputs=9
  Demux2 : Demux  Outputs=9
  FA1 : Subsystem
  FA10 : Subsystem
  FA2 : Subsystem
  FA3 : Subsystem
  FA4 : Subsystem
  FA5 : Subsystem
  FA6 : Subsystem
  FA7 : Subsystem
  FA9 : Subsystem
  NOT : Logic  Operator=NOT  IconShape=distinctive  AllPortsSameDT=off  OutDataTypeStr=boolean
  Terminator{1..9} (9 alike) : Terminator
  a < b : Outport
  wires:
  FA7/2(Co) -> FA6/3(Cin)
  FA6/2(Co) -> FA5/3(Cin)
  FA5/2(Co) -> FA4/3(Cin)
  FA4/2(Co) -> FA3/3(Cin)
  FA3/2(Co) -> FA2/3(Cin)
  FA2/2(Co) -> FA1/3(Cin)
  FA9/2(Co) -> FA7/3(Cin)
  FA10/2(Co) -> FA9/2(Cin)
  Constant/1 -> FA10/3(Cin)
  FA1/2(Co) -> Terminator2/1
  Demux1/9 -> FA10/1(B0)
  Demux1/8 -> FA9/1(B0)
  Demux1/7 -> FA7/1(B0)
  Demux1/6 -> FA6/1(B0)
  Demux1/5 -> FA5/1(B0)
  Demux1/4 -> FA4/1(B0)
  Demux1/2 -> FA2/1(B0)
  Demux1/3 -> FA3/1(B0)
  Demux1/1 -> FA1/1(B0)
  FA1/1(S) -> a < b/1
  Demux2/5 -> FA5/2(B1)
  Demux2/6 -> FA6/2(B1)
  Demux2/1 -> FA1/2(B1)
  Demux2/3 -> FA3/2(B1)
  Demux2/4 -> FA4/2(B1)
  Demux2/2 -> FA2/2(B1)
  Demux2/7 -> FA7/2(B1)
  Demux2/9 -> FA10/2(B1)
  Demux2/8 -> FA9/3(B1)
  FA2/1(S) -> Terminator1/1
  FA3/1(S) -> Terminator3/1
  FA4/1(S) -> Terminator4/1
  FA5/1(S) -> Terminator5/1
  FA6/1(S) -> Terminator6/1
  FA7/1(S) -> Terminator7/1
  FA9/1(S) -> Terminator8/1
  FA10/1(S) -> Terminator9/1
  b/1 -> NOT/1
  a/1 -> Demux1/1
  NOT/1 -> Demux2/1
